simulink model "RobotX_ss_acousticsSingle_Dock_LB_ODOA_23commQualRun4pm_1025"  (R2014a)
settings: Solver=FixedStepDiscrete  StartTime=0.0  StopTime=inf  FixedStep=.25  RelTol=1e-3
undefined symbols (not defined in the file): Com1, Com2, Com3, Com4, DiscIntNeverNeededParam, standard
libraries: xpcseriallib x42, simulink x19, slrtlib x7, dspmtrx3 x2, speedgoatlib x2, speedgoatlib_IO102 x1
(part 5 of 7)

== matlab function RobotX_ss_acousticsSingle_Dock_LB_ODOA_23commQualRun4pm_1025/Main FSM/LightTower/MATLAB Function ==
  data: ltTask input; taskSelector output; pointFin input; foundInPoint input; cornerFin input; turnForSweepFin input; sweepFin input; turnForApproachFin input; approachFin input; sequenceFin input; pointEn output; cornerEn output; turnForSweepEn output; sweepEn output; turnForApproachEn output; approachEn output; sequenceEn output; reportEn output
function  [taskSelector, pointEn, cornerEn, turnForSweepEn, sweepEn, turnForApproachEn, approachEn, ...
    sequenceEn, reportEn]= ltEnabler(ltTask, pointFin, foundInPoint, ...
    cornerFin, turnForSweepFin, sweepFin, turnForApproachFin, approachFin, sequenceFin)

%%  Written by Michael Benson on October 23, 2014
%   Changes the value of ltTask and the enablers for the tasks within the
%   light tower task FSM.

%% Initialize enable signals
pointEn = 0;
cornerEn = 0;
turnForSweepEn = 0;
sweepEn = 0;
turnForApproachEn = 0;
approachEn = 0;
sequenceEn = 0;
reportEn = 0;

%% Adjust finished states based on user task selection
ltTaskStr = char(ltTask);

if ~isempty(strfind(ltTaskStr,'corner'))
    pointFin = 1;
elseif ~isempty(strfind(ltTaskStr,'sweep'))
    pointFin = 1;
    cornerFin = 1;
    turnForSweepFin = 1;
elseif ~isempty(strfind(ltTaskStr,'approach'))
    pointFin = 1;
    cornerFin = 1;
    turnForSweepFin = 1;
    sweepFin = 1;
elseif ~isempty(strfind(ltTaskStr,'sequence'))
    pointFin = 1;
    cornerFin = 1;
    turnForSweepFin = 1;
    sweepFin = 1;
    turnForApproachFin = 1;
    approachFin = 1;
elseif ~isempty(strfind(ltTaskStr,'report'))
    pointFin = 1;
    cornerFin = 1;
    turnForSweepFin = 1;
    sweepFin = 1;
    turnForApproachFin = 1;
    approachFin = 1;
    sequenceFin = 1;
end

if foundInPoint == 1
    pointFin = 1;
    cornerFin = 1;
    turnForSweepFin = 1;
    sweepFin = 1;
end
    

%% Set enable signals based on state completion
if pointFin == 0
    pointEn = 1;
    taskSelector = 1;
elseif cornerFin == 0
    cornerEn = 1;
    taskSelector = 2;
elseif turnForSweepFin == 0
    turnForSweepEn = 1;
    taskSelector = 3;
elseif sweepFin == 0
    sweepEn = 1;
    taskSelector = 4;
elseif turnForApproachFin == 0
    turnForApproachEn = 1;
    taskSelector = 5;
elseif approachFin == 0
    approachEn = 1;
    taskSelector = 6;
elseif sequenceFin == 0
    sequenceEn = 1;
    taskSelector = 7;
else
    reportEn = 1;
    taskSelector = 8;
end

== matlab function RobotX_ss_acousticsSingle_Dock_LB_ODOA_23commQualRun4pm_1025/Sensors/1025 Comms New LIDAR Mode/Message Selector/HRTLIT Message/MATLAB Function1 ==
  data: ltSeq input; LITValid output; LITSequence output
function [LITValid,LITSequence] = LITSeqParse(ltSeq)

LITValid = ltSeq(1);
LITSequence = ltSeq(2:4);

== matlab function RobotX_ss_acousticsSingle_Dock_LB_ODOA_23commQualRun4pm_1025/Sensors/1025 Comms New LIDAR Mode/Pi Nav Send/Data Update2 ==
  data: Valid input; ControlMode input; V output; C output; L output; A output; Data input; D1 output; D2 output; D3 output; D4 output; D5 output; D6 output; D7 output; D8 output; D9 output; D10 output; D11 output; D12 output; D13 output; D14 output; D15 output; D16 output; D17 output; D18 output; D19 output; D20 output; D21 output; D22 output; D23 output; D24 output; Activate input
function [V,C,L,A,D1,D2,D3,D4,D5,D6,D7,D8,D9,D10,D11,D12,D13,D14,D15,D16,D17,...
    D18,D19,D20,D21,D22,D23,D24] = dataSplit(Valid,ControlMode,Data,Activate)
%Written by Anderson Lebbad on August 10, 2014
%Last Edited by: Anderson Lebbad on September 11, 2014

%This function splits the data vector into the twelve channels it is
%composed of for communication

persistent HoldData

if isempty(HoldData)
    HoldData = zeros(26,1);
    HoldData(2) = 2;
end

if Valid == 1
    HoldData(1) = Valid;
    HoldData(2) = ControlMode;
    HoldData(3) = Data(1);
    HoldData(4) = Data(2);
    HoldData(5) = Data(3);
    HoldData(6) = Data(4);
    HoldData(7) = Data(5);
    HoldData(8) = Data(6);
    HoldData(9) = Data(7);
    HoldData(10) = Data(8);
    HoldData(11) = Data(9);
    HoldData(12) = Data(10);
    HoldData(13) = Data(11);
    HoldData(14) = Data(12);
    HoldData(15) = Data(13);
    HoldData(16) = Data(14);
    HoldData(17) = Data(15);
    HoldData(18) = Data(16);
    HoldData(19) = Data(17);
    HoldData(20) = Data(18);
    HoldData(21) = Data(19);
    HoldData(22) = Data(20);
    HoldData(23) = Data(21);
    HoldData(24) = Data(22);
    HoldData(25) = Data(23);
    HoldData(26) = Data(24);
end

V = HoldData(1);
C = HoldData(2);
L = 8;
A = Activate;
D1 = HoldData(3);
D2 = HoldData(4);
D3 = HoldData(5);
D4 = HoldData(6);
D5 = HoldData(7);
D6 = HoldData(8);
D7 = HoldData(9);
D8 = HoldData(10);
D9 = HoldData(11);
D10 = HoldData(12);
D11 = HoldData(13);
D12 = HoldData(14);
D13 = HoldData(15);
D14 = HoldData(16);
D15 = HoldData(17);
D16 = HoldData(18);
D17 = HoldData(19);
D18 = HoldData(20);
D19 = HoldData(21);
D20 = HoldData(22);
D21 = HoldData(23);
D22 = HoldData(24);
D23 = HoldData(25);
D24 = HoldData(26);

end

== matlab function RobotX_ss_acousticsSingle_Dock_LB_ODOA_23commQualRun4pm_1025/Main FSM/Docking/Docking/MATLAB Function ==
  data: QuayHeading input; TargetPoints input; Finished output; X input; Data output; Y input; Psi input; Dist input; Angles input; Prob input; Time input; dockNum input
function [Finished,Data] = Orient(QuayHeading,TargetPoints,X,Y,Psi,Dist,Angles,Prob,Time,dockNum)
%Written by Dylan DeGaetano on September 2, 2014
%Last Edited By Anderson Lebbad on September 19 2014

%This function passes the current pose data with the requrested heading
%so that the boat is facing the Quay wall.This task must be in station
%keeping mode
%
%Anderson's edit moved the orient within this function and adjusts the code
%to work better with sensing information

% 10/21 Edit: Correlates the estimated NED coord of the found symbol with
% known locations found through Ivan's map and proceeds to those locations

% Input TargetPoint is a 10x2 matrix of NED coords structured as follows
% [Observation Point; Dock1Start; Dock1Inter; Dock1Fin; Dock2Start;
% Dock2Inter; Dock2Fin; Dock3Start; Dock3Inter; Dock3Fin] where the bay
% numbers go from left to right

%work aound for communication issue
idx = Prob(4);
% Holdpose = station keeping point that we want to get to
% Pose = which waypoint to head to
% posIdx = which docking symbol position it is @
% 1 = Left, 2 = Middle, 3 = Right
% recognized = flag for if position of dock is found

persistent holdPose pos posIdx recognized

% If not to hold position
if isempty(holdPose)
    holdPose = [TargetPoints(1,:) QuayHeading]; % Initialize with Observation Points
    pos = 0;
    posIdx = 0;
    recognized = 0;
end

DistM=Dist(1)/100; % CM to M
Finished = 0; % Task not completed

%Initialize Data variable
Data = zeros(24,1); % 24x1 Array of Zeros


if idx(1) ~= 0 && recognized == 0
    %Calculate the NED coordinate of the found symbol
    TargetX = X+DistM(idx(1))*cos((Psi+Angles(idx(1)))*pi/180);
    TargetY = Y+DistM(idx(1))*sin((Psi+Angles(idx(1)))*pi/180);
    
    % Since the quay wall is very well aligned with EW directions,
    % correlate the estimated E coord of the found symbol with one of
    % the known bay positions
    bayEPos = [TargetPoints(4,2); TargetPoints(7,2); TargetPoints(10,2)];
    PosDiff = bayEPos - TargetY;
    [~,posIdx] = min(PosDiff);
    
    % Flag symbol as recognized
    recognized = 1; % Ensure that this calculation is not made again after the dock symbol pos is found/calculated
    
    % Begin proceeding to first position
    pos = 1;
end

if pos == 1
        %Set destination in front of dock to line up
        holdPose(1) = TargetPoints(pos+posIdx+2^(posIdx-1),1); % North
        holdPose(2) = TargetPoints(pos+posIdx+2^(posIdx-1),2); % East
    
    l1norm = abs(X-holdPose(1))+abs(Y-holdPose(2)); % calculate range to point we want to get to
    
    if l1norm < 2 % 2 metters
        % If within range, then flag first position complete and begin
        % proceeding to the hext position
        pos = 2;
    end
elseif pos == 2
        % Set intermediate point between start and finish
        holdPose(1) = TargetPoints(pos+posIdx+2^(posIdx-1),1); % North
        holdPose(2) = TargetPoints(pos+posIdx+2^(posIdx-1),2); % East
    
    l2norm = abs(X-holdPose(1)) + abs(Y-holdPose(2));
    
    if l2norm < 2
        % If within range, then flag second position complete and begin
        % proceeding to the hext position
        pos = 3;
    end
elseif pos == 3
        % Set final docking point
        holdPose(1) = TargetPoints(pos+posIdx+2^(posIdx-1),1); % North
        holdPose(2) = TargetPoints(pos+posIdx+2^(posIdx-1),2); % East
    
    l3norm = abs(X-holdPose(1)) + abs(Y-holdPose(2));
    
    if l3norm < 2
        holdPose = [X Y QuayHeading];
        Finished = 1;
    end
end

if Time >= 120 && recognized == 0
    % If symbol cannot be found within 60 seconds, proceed to middle bay
    posIdx = dockNum;
    recognized = 1;
end

holdPose(3) = QuayHeading;

Data(1) = holdPose(1);
Data(2) = holdPose(2);
Data(3) = holdPose(3);

== matlab function RobotX_ss_acousticsSingle_Dock_LB_ODOA_23commQualRun4pm_1025/Sensors/1020 Comms/MATLAB Function2 ==
  data: Time input; asciiLIT output; Sequence input
% This function creates the light tower message to be sent from 
% Speedgoat in ascii code
% Written by: Edward Zhu
% Date: 9/17/14

function asciiLIT = asciiLITEncoder(Time, Sequence)

% Initialize output message vector as the serial output block expects 128
% character message
asciiLIT = uint8(zeros(1,128));

% Convert static strings to ascii code
asciiMsgID = uint8('$RXLIT,');
asciiComma = uint8(',');
asciiTeamID = uint8('FAUVU,');
asciiMsgEnd = uint8('*');
asciiMsgCRLF = [13 10];

% Convert UTC Time input (hhmmss) into ascii code
asciiTime = uint8(zeros(1,7));
asciiTime(7) = asciiComma;

for timeChar = 1:6
    asciiTime(timeChar) = floor(mod(Time,10^(7-timeChar))/...
        10^(6-timeChar)) + 48;
end

% Convert the light sequece into ascii code (1 = R, 2 = B, 3 = G)
asciiSeq = uint8(zeros(1,4)+32);
asciiSeq(4) = asciiMsgEnd;

if Sequence(1) > 0 && Sequence(2) > 0 && Sequence(3) > 0
    for seqChar = 1:3
        if Sequence(seqChar) == 1
            Sequence(seqChar) = uint8('R');
        elseif Sequence(seqChar) == 2
            Sequence(seqChar) = uint8('B');
        elseif Sequence(seqChar) == 3
            Sequence(seqChar) = uint8('G');
        end
    end
    asciiSeq(1:3) = Sequence;
end

% Concat individual ascii arrays into one array
asciiPreChkSum = cat(2,asciiMsgID,asciiTime,asciiTeamID,asciiSeq);

% Calculate the checksum of the message from the '$' to the '*' and convert
% to hex
chkSum = uint8(0);

for chksumChar = 1:(length(asciiPreChkSum)-2)
    chkSum = bitxor(chkSum,asciiPreChkSum(chksumChar+1));
end

% Convert the checksum to ascii
chkSum = dec2hex(chkSum);
asciiChkSum = uint8(zeros(1,length(chkSum))+32);
for i = 1:length(chkSum)
    asciiChkSum(i) = uint8(chkSum(i));
end

% Concat the checksum and the '/r/n' to the end of the message
asciiPostChkSum = cat(2,asciiPreChkSum,asciiChkSum,asciiMsgCRLF);

% Output the final message
asciiLIT(1:length(asciiPostChkSum)) = asciiPostChkSum;

== matlab function RobotX_ss_acousticsSingle_Dock_LB_ODOA_23commQualRun4pm_1025/Main FSM/LightTower/Sweep Field/Spin, Listen, and Point/Look for Light Tower ==
  data: subsetCorners input; X input; Y input; Psi input; Distances input; Angles input; Data output; Finished output; FoundTower output; TowerLoc output; spinAmount input
function [Data, Finished, FoundTower, TowerLoc] = fcn(...
    subsetCorners, X, Y, Psi, Distances, Angles, spinAmount)

%   Written by Michael Benson on October 23, 2014
%   This function spins the WAM-V to look for the light tower.  If it
%   sees an object, and that object is within the field subset, the boat
%   will hold pose and the Lidar will continue to evaluate an object.  If
%   the object is still there within that time, it determines that that
%   object is the buoy and ends the task.  Otherwise, the task exits
%   without setting FoundTower high.

[Distances,I] = sort(Distances);
Angles = Angles(I);

persistent FoundHeading FoundCounter desiredHeading initHeading minPose maxPose minReached maxReached

offset = 5;

if isempty(FoundHeading) && isempty(FoundCounter) && isempty(desiredHeading) && isempty(initHeading) && isempty(minReached) && isempty(maxReached)
    FoundCounter = 0;
    minPose = Psi - spinAmount/2;
    maxPose = Psi + spinAmount/2;
    minReached = 0;
    maxReached = 0;
    initHeading = Psi;
    desiredHeading = Psi+offset;
    FoundHeading = 0;
end

Finished = 0;
FoundTower = 0;
Data = zeros(24,1);
TowerLoc = zeros(1,2);
LandmarkLocations = zeros(12,2);
LandmarkDistances = zeros(12,1);

ObjectInfo = [Distances,Angles];


%% Landmark Analysis
if ObjectInfo(12,1) ~= 0 && ObjectInfo(12,2) ~= 0
    %calculate location of each landmark and determine if it is in the
    %bounding box
    for i = 12-sum(Distances ~= 0)+1:12
        LandmarkX = X + cos((Psi+Angles(i))*pi/180)*Distances(i)/100;
        LandmarkY = Y + sin((Psi+Angles(i))*pi/180)*Distances(i)/100;
        LandmarkValid = inBbox(subsetCorners,[LandmarkX LandmarkY]);
        if LandmarkValid == 1
            LandmarkLocations(i,1:2) = [LandmarkX LandmarkY];
            LandmarkDistances(i) = Distances(i);
        end
    end
    
    [~,I] = sort(LandmarkDistances);
    LandmarkLocations = LandmarkLocations(I);
    
    if sum(LandmarkDistances ~= 0) >= 1
        FoundTower = 1;
        TowerLoc = LandmarkLocations(12-sum(LandmarkDistances ~= 0)+1,1:2);
        FoundCounter = FoundCounter + 1;
        if FoundCounter == 1;
            FoundHeading = Psi;
        end
        desiredHeading = FoundHeading;
    end
else
    FoundCounter = 0;
    if abs(Psi-maxPose) < 5
        maxReached = 1;
    elseif abs(Psi-minPose) < 5
        minReached = 1;
    end
    
    if maxReached == 1
        desiredHeading = Psi - offset;
    elseif maxReached == 1 && minReached == 1
        desiredHeading = initHeading;
        Finished = 1;
    end
end

Data(1:3) = [X Y desiredHeading];

end

function [ inBbox ] = inBbox( bbox, point )
%UNTITLED Summary of this function goes here
%   Detailed explanation goes here
b1 = bbox(1,:);
b2 = bbox(2,:);
b3 = bbox(3,:);
b4 = bbox(4,:);

t1 = inTriangle(point,b1,b2,b3);
t2 = inTriangle(point,b1,b2,b4);
t3 = inTriangle(point,b1,b3,b4);

if t1 && t2 && t3
    inBbox = 1;
else
    inBbox = 0;
end

end

function [ inTri ] = inTriangle(p, a, b, c)

s1 = sameSide(p,a,b,c);
s2 = sameSide(p,b,a,c);
s3 = sameSide(p,c,a,b);

if s1 || s2 || s3
    inTri = 1;
else
    inTri = 0;
end

end

function [ onSame ] = sameSide(p1,p2,a,b)

theta = atan2(b(2)-a(2),b(1)-a(1));
R = [cos(theta), sin(theta); -sin(theta), cos(theta)];
side1 = R*(p1-a)';
side2 = R*(p2-a)';
same = side1(2)/side2(2);
onSame = same >= 0;

end

== matlab function RobotX_ss_acousticsSingle_Dock_LB_ODOA_23commQualRun4pm_1025/Main FSM/LightTower/Turn For Sweep/LLA to NED ==
  data: GoalLLA input; GoalNED output; NED_origin input
function GoalNED = LLA2NEDfun(GoalLLA,NED_origin)
%Written by Anderson Lebbad on September 20, 2014
%Last edited by:
%
%This function converts a target Latitude, Longitude, Altitude (LLA) point
%into North, East, Down (NED) coordinates
GoalNED = zeros(size(GoalLLA));
for i = 1:size(GoalLLA,1)
    %First convert to earth centered, earth fixed frame
    GoalECEF = lla2ecef([GoalLLA(1)*(pi/180), GoalLLA(2)*(pi/180), 0]');
    %Then convert from ECEF to North East Down
    GoalNEDvect = ecef2ned([NED_origin(1)*(pi/180),NED_origin(2)*(pi/180)],GoalECEF);
    GoalNED(i,:) = GoalNEDvect(1:2)';
end

end

function x_ecef = lla2ecef(x_lla)
% LLE2ECEF: Converts from geodetic latitude, longitude, and altitude to earth-centered earth-fixed Cartesian coordinates
% INPUT: latitude phi (rad), longitude lambda (rad), altitude h (m)
% OUTPUT: [x, y, z]' (m) earth-centered earth-fixed Cartesian coordinates
    a = 6378137; % equatorial radius of ellipsoid (semi-major axis) (m)
    b = 6356752; % polar axis radius of ellipsoid (semi-minor axis) (m)

    phi = x_lla(1);
    lambda = x_lla(2);
    h = x_lla(3);
    
    % auxiliar quantities f, e, and N
    f = (a-b)/a;
    e = f*(2-f);
    N = a/sqrt(1-(e*sin(phi))^2);
    x_ecef = [(N+h)*cos(phi)*cos(lambda); (N+h)*cos(phi)*sin(lambda); (N*(1-e^2)+h)*sin(phi)];
end

function [x_ned] = ecef2ned(ned_lla, x_ecef)
% ECEF2NED Converts from earth-centered, earth-fixed Cartesian coordinates to tangent plane
% INPUT:
% 1) x_ecef=[x,y,z]' (m) earth-centered, earth-fixed Cartesian coordinates
% 2) ned_lla=[phi,lambda]' consiting of latitude phi (rad), longitude lambda (rad) of NED origin
% OUTPUT:
% 1) x_ned=[x,y,z]' (m) in NED coordinate system with the origin [phi,lambda]'

    phi = ned_lla(1);
    lambda = ned_lla(2);

    % transformation  matrix
    T = [-sin(phi)*cos(lambda) -sin(phi)*sin(lambda)  cos(phi)
         -sin(lambda)           cos(lambda)           0
          cos(phi)*cos(lambda)   cos(phi)*sin(lambda)  sin(phi)];

     x_ned = T*(x_ecef-lla2ecef([phi, lambda, 0]')); % convert to NED
     x_ned(3) = -x_ned(3);
end

== matlab function RobotX_ss_acousticsSingle_Dock_LB_ODOA_23commQualRun4pm_1025/Main FSM/ODOA/Entry Gate/Entry Gate Align/MATLAB Function1 ==
  data: EnterGateNED input; entryNED output; gateNumber input
function entryNED = EntryGPSSelector(EnterGateNED,gateNumber)

entryNED = EnterGateNED(gateNumber,:);

== matlab function RobotX_ss_acousticsSingle_Dock_LB_ODOA_23commQualRun4pm_1025/Main FSM/ODOA/Entry Gate/Entry Gate Enabler ==
  data: StartFin input; TaskSelector output; StartEn output; AlignFin input; AlignEn output; ThroughEn output
function [TaskSelector, StartEn,AlignEn,ThroughEn] = entryGateEnabler(StartFin, AlignFin)

StartEn = 0;
AlignEn = 0;
ThroughEn = 0;

if StartFin == 0
    StartEn = 1;
    TaskSelector = 1;
elseif AlignFin == 0
    AlignEn = 1;
    TaskSelector = 2;
else
    ThroughEn = 1;
    TaskSelector = 3;
end

== matlab function RobotX_ss_acousticsSingle_Dock_LB_ODOA_23commQualRun4pm_1025/Main FSM/ODOA/Entry Gate/Entry Gate Through/CalcTimes ==
  data: pts input; u input; Data output
function Data = calcTimes(pts, u)
%Written by Anderson Lebbad on August 9, 2014
%Last Edited: Dylan DeGaetano September 1, 2014

%Calculates times for the boat to get to points for a trajectory, and
%formats Data for communication

%Initialize
Data = zeros(24,1);
traj = zeros(8,3);
traj(:,1:2) = pts;



for k = 2:8
    %Calculate distance to travel from last point
    distTravel = sqrt(sum((pts(k-1,:)-pts(k,:)).^2));
    %Assume 1m per second speed
    traj(k,3) = traj(k-1,3) + distTravel;
    %Add time based off initial velocity to get to first point past initial
    if k == 2
        traj(k,3) = traj(k,3) + 2.5*abs(2-u);
    end
end


%Output Data
for i=1:8
    for j = 1:3
        Data(3*(i-1)+j) = traj(i,j);
    end
end

== matlab function RobotX_ss_acousticsSingle_Dock_LB_ODOA_23commQualRun4pm_1025/Main FSM/ODOA/Entry Gate/Entry Gate Through/MATLAB Function ==
  data: dist input; X input; Y input; Psi input; GoalNED output
function GoalNED = travelAlongHeading(dist, X, Y, Psi)
%Written by Michael Benson on October 23, 2014

%This function determines the target NED point for the Sweep Field subtask
%for the Light Tower task.  The target point is Distance meters from the
%current ASV position, and is towards the opposite corner of the subset
%field.

persistent lockedHeading

Psi = Psi*180/pi;

if isempty(lockedHeading)
    lockedHeading = Psi;
end

GoalNED = [X+dist*cos(lockedHeading*pi/180) Y+dist*sin(lockedHeading*pi/180)];

== matlab function RobotX_ss_acousticsSingle_Dock_LB_ODOA_23commQualRun4pm_1025/Main FSM/ODOA/Entry Gate/GPS Move/GPSMove ==
  data: GoalNED input; X input; Finished output; valid output; Y input; Psi input; pts output
function [Finished,valid,pts] = GPSmove(GoalNED,X,Y,Psi)
%Written by Dylan DeGaetano on September 1, 2014
%Last edited by: Anderson Lebbad
%
%This function will go to a given NED cooridnate, last edit changed the
%goal pt and variable names

% Input of GoalNED is a 10x2 matrix of NED coords where the first row is
% the coord of the docking observation point

persistent Sample
if isempty(Sample)
Sample = 0;
end
Finished = 0;
pts = zeros(8,2);
%$Distance to object in meters
if Sample == 100
    Sample = 0;
end

if Sample == 0
    pts(1,1) = X+5*cos(Psi*pi/180);
    pts(1,2) = Y+5*sin(Psi*pi/180);
    pts(8,1) = GoalNED(1,1);
    pts(8,2) = GoalNED(1,2);
    pts(2,:) = pts(1,:) +(1*(GoalNED(1,:)-pts(1,:))/7);
    pts(3,:) = pts(1,:) +(2*(GoalNED(1,:)-pts(1,:))/7);
    pts(4,:) = pts(1,:) +(3*(GoalNED(1,:)-pts(1,:))/7);
    pts(5,:) = pts(1,:) +(4*(GoalNED(1,:)-pts(1,:))/7);
    pts(6,:) = pts(1,:) +(5*(GoalNED(1,:)-pts(1,:))/7);
    pts(7,:) = pts(1,:) +(6*(GoalNED(1,:)-pts(1,:))/7);
    Sample = 1; 
    valid = 1;
    
else 
    range = sqrt(sum((GoalNED(1,:) - [X Y]).^2));
    if range <= 5
        Finished = 1;
    end
    valid = 0;
    Sample = Sample + 1;
end

== matlab function RobotX_ss_acousticsSingle_Dock_LB_ODOA_23commQualRun4pm_1025/Main FSM/ODOA/Exit Gate/Exit Gate Through/MATLAB Function ==
  data: dist input; X input; Y input; Psi input; GoalNED output
function GoalNED = travelAlongHeading(dist, X, Y, Psi)
%Written by Michael Benson on October 23, 2014

%This function determines the target NED point for the Sweep Field subtask
%for the Light Tower task.  The target point is Distance meters from the
%current ASV position, and is towards the opposite corner of the subset
%field.

persistent lockedHeading

Psi = Psi*180/pi;

if isempty(lockedHeading)
    lockedHeading = Psi;
end

GoalNED = [X+dist*cos(lockedHeading*pi/180) Y+dist*sin(lockedHeading*pi/180)];

== matlab function RobotX_ss_acousticsSingle_Dock_LB_ODOA_23commQualRun4pm_1025/Main FSM/ODOA/GPS Beeline/GPSMove ==
  data: dodgeStart output; GoalNED input; X input; Finished output; valid output; Y input; Psi input; pts output; Distances input
function [dodgeStart,Finished,valid,pts] = GPSmove(GoalNED,X,Y,Psi,Distances)
%Written by Dylan DeGaetano on September 1, 2014
%Last edited by: Anderson Lebbad
%
%This function will go to a given NED cooridnate, last edit changed the
%goal pt and variable names

% Input of GoalNED is a 10x2 matrix of NED coords where the first row is
% the coord of the docking observation point

DistM = Distances/100;

DistM = sort(DistM);
dodgeStart = 0;

persistent Sample
if isempty(Sample)
Sample = 0;
end
Finished = 0;
pts = zeros(8,2);
%$Distance to object in meters
if Sample == 100
    Sample = 0;
end

if Sample == 0
    pts(1,1) = X+5*cos(Psi*pi/180);
    pts(1,2) = Y+5*sin(Psi*pi/180);
    pts(8,1) = GoalNED(1,1);
    pts(8,2) = GoalNED(1,2);
    pts(2,:) = pts(1,:) +(1*(GoalNED(1,:)-pts(1,:))/7);
    pts(3,:) = pts(1,:) +(2*(GoalNED(1,:)-pts(1,:))/7);
    pts(4,:) = pts(1,:) +(3*(GoalNED(1,:)-pts(1,:))/7);
    pts(5,:) = pts(1,:) +(4*(GoalNED(1,:)-pts(1,:))/7);
    pts(6,:) = pts(1,:) +(5*(GoalNED(1,:)-pts(1,:))/7);
    pts(7,:) = pts(1,:) +(6*(GoalNED(1,:)-pts(1,:))/7);
    Sample = 1; 
    valid = 1;
    
else 
    range = sqrt(sum((GoalNED(1,:) - [X Y]).^2));
    if range <= 5
        Finished = 1;
    end
    valid = 0;
    Sample = Sample + 1;
end

if sum(DistM ~= 0) > 0
    closestRange = DistM(12-sum(DistM ~= 0)+1);
    if closestRange < 10
        dodgeStart = 1;
    end
end

== matlab function RobotX_ss_acousticsSingle_Dock_LB_ODOA_23commQualRun4pm_1025/Main FSM/Start//Speedgate/GPS Move/CalcTimes ==
  data: pts input; u input; Data output
function Data = calcTimes(pts, u)
%Written by Anderson Lebbad on August 9, 2014
%Last Edited: Dylan DeGaetano September 1, 2014

%Calculates times for the boat to get to points for a trajectory, and
%formats Data for communication

%Initialize
Data = zeros(24,1);
traj = zeros(8,3);
traj(:,1:2) = pts;



for k = 2:8
    %Calculate distance to travel from last point
    distTravel = sqrt(sum((pts(k-1,:)-pts(k,:)).^2));
    %Assume 1m per second speed
    traj(k,3) = traj(k-1,3) + distTravel;
    %Add time based off initial velocity to get to first point past initial
    if k == 2
        traj(k,3) = traj(k,3) + 2.5*abs(2-u);
    end
end


%Output Data
for i=1:8
    for j = 1:3
        Data(3*(i-1)+j) = traj(i,j);
    end
end

== matlab function RobotX_ss_acousticsSingle_Dock_LB_ODOA_23commQualRun4pm_1025/Main FSM/Start//Speedgate/Main Enabler ==
  data: taskSelector output; GpsEn output; entEn output; exitEn output; ssgateTask input; GpsFin input; entFin input
function [taskSelector,GpsEn,entEn,exitEn]=Startgate_Enabler(ssgateTask,...
    GpsFin,entFin)
%Written by Anderson Lebbad on July 19, 2013
%Last Edited: Dylan DeGaetano on September ,4 2014
%   Substring search for task was written in
%   Case switches were redundant, combined with first set of if statements

%Changes the value of MainMode and the enablers for the tasks within the
%Main FSM.

% Initialize enable signals
GpsEn = 0;
entEn =0;
exitEn = 0;

% Convert main task indicator to a string
ssgateTaskStr = char(ssgateTask);

% Adjust finished states based on user task selection (never skips
% initialization)
if ~isempty(strfind(ssgateTaskStr,'Aim'))
    GpsFin = 1;
elseif ~isempty(strfind(ssgateTaskStr,'Start'))
    GpsFin = 1;
    entFin = 1;
elseif ~isempty(strfind(ssgateTaskStr,'Speed'))
    GpsFin = 1;
    entFin = 1;
end

% Set enable signals based on state completion
if GpsFin == 0
    GpsEn = 1;
    taskSelector = 1;
elseif entFin == 0
    entEn = 1;
    taskSelector = 2;
else
    exitEn = 1;
    taskSelector = 3;
end

== system RobotX_ss_acousticsSingle_Dock_LB_ODOA_23commQualRun4pm_1025/Main FSM/ODOA/Entry Gate/Entry Gate Align ==
  Sensors : Inport
  Enable : EnablePort  ShowOutputPort=on
  Bus Selector : BusSelector  OutputSignals=Navigation Message.Pose.X,Navigation Message.Pose.Y,Navigation Message.Pose.Psi,Lidar Data Input.Landmarks.Distances,Lidar Data Input.Landmarks.Angles
  Compare To Constant : simulink/Logic and Bit Operations/Compare To Constant  relop=>=  const=120  OutDataTypeStr=boolean
  Data Store Read : DataStoreRead  DataStoreName=EnterGateNED
  Data Store Read1 : DataStoreRead  DataStoreName=ODOAentry
  Data Store Read2 : DataStoreRead  DataStoreName=QuayHeading
  Data Store Read3 : DataStoreRead  DataStoreName=ODOAstartNED
  Data Type Conversion : DataTypeConversion  OutDataTypeStr=double
  Discrete-Time Integrator : DiscreteIntegrator  SampleTime=-1  ICPrevOutput=DiscIntNeverNeededParam  ICPrevScaledInput=DiscIntNeverNeededParam
  Logical Operator : Logic  Operator=OR  AllPortsSameDT=off  OutDataTypeStr=boolean
  MATLAB Function : MATLAB Function  TreatAsAtomicUnit=on
  MATLAB Function1 : MATLAB Function  TreatAsAtomicUnit=on
  Output Heirarchy : Subsystem
  Outputs : Outport
  Finished : Outport  Port=2
  wires:
  Output Heirarchy/1(Outputs) -> Outputs/1
  Sensors/1 -> Output Heirarchy/2(Sensors), Bus Selector/1
  Data Store Read1/1 -> MATLAB Function1/2(gateNumber)
  Data Store Read/1 -> MATLAB Function1/1(EnterGateNED)
  MATLAB Function1/1(entryNED) -> MATLAB Function/1(entryNED)
  Bus Selector/1 -> MATLAB Function/5(X)  "<X>"
  Bus Selector/5 -> MATLAB Function/9(Angles)  "<Angles>"
  Bus Selector/2 -> MATLAB Function/6(Y)  "<Y>"
  Bus Selector/4 -> MATLAB Function/8(Distances)  "<Distances>"
  Bus Selector/3 -> MATLAB Function/7(Psi)  "<Psi>"
  MATLAB Function/2(Finished) -> Logical Operator/1
  MATLAB Function/1(Data) -> Output Heirarchy/1(Data)
  Discrete-Time Integrator/1 -> Compare To Constant/1, MATLAB Function/4(Time)
  Enable/1 -> Discrete-Time Integrator/1
  Data Store Read2/1 -> MATLAB Function/3(QuayHeading)
  Data Store Read3/1 -> MATLAB Function/2(startNED)
  Compare To Constant/1 -> Logical Operator/2
  Logical Operator/1 -> Data Type Conversion/1
  Data Type Conversion/1 -> Finished/1

== system RobotX_ss_acousticsSingle_Dock_LB_ODOA_23commQualRun4pm_1025/Main FSM/ODOA/Entry Gate/Entry Gate Through ==
  Sensors : Inport
  Enable : EnablePort
  Bus Selector : BusSelector  OutputSignals=Navigation Message.Pose.X,Navigation Message.Pose.Y,Navigation Message.Pose.Psi,Navigation Message.Velocity.u
  CalcTimes : MATLAB Function  TreatAsAtomicUnit=on
  Distance to Travel : Constant  Value=15
  GPSMove : MATLAB Function  TreatAsAtomicUnit=on
  MATLAB Function : MATLAB Function  TreatAsAtomicUnit=on
  Output Reassign : Subsystem
  Outputs : Outport
  Finished : Outport  Port=2
  wires:
  GPSMove/3(pts) -> CalcTimes/1(pts)
  Sensors/1 -> Output Reassign/3(Sensors), Bus Selector/1
  Bus Selector/1 -> MATLAB Function/2(X), GPSMove/2(X)  "<X>"
  Bus Selector/2 -> MATLAB Function/3(Y), GPSMove/3(Y)  "<Y>"
  Bus Selector/3 -> MATLAB Function/4(Psi), GPSMove/4(Psi)  "<Psi>"
  Bus Selector/4 -> CalcTimes/2(u)  "<u>"
  GPSMove/1(Finished) -> Finished/1
  Output Reassign/1(Outputs) -> Outputs/1
  CalcTimes/1(Data) -> Output Reassign/2(Data)
  GPSMove/2(valid) -> Output Reassign/1(Vaild)
  MATLAB Function/1(GoalNED) -> GPSMove/1(GoalNED)
  Distance to Travel/1 -> MATLAB Function/1(dist)

== system RobotX_ss_acousticsSingle_Dock_LB_ODOA_23commQualRun4pm_1025/Main FSM/ODOA/Entry Gate/GPS Move ==
  Sensors : Inport
  Enable : EnablePort
  Bus Selector : BusSelector  OutputSignals=Navigation Message.Pose.X,Navigation Message.Pose.Y,Navigation Message.Pose.Psi,Navigation Message.Velocity.u
  CalcTimes : MATLAB Function  TreatAsAtomicUnit=on
  Data Store Read : DataStoreRead  DataStoreName=EnterGateNED
  Data Store Read1 : DataStoreRead  DataStoreName=ODOAentry
  GPSMove : MATLAB Function  TreatAsAtomicUnit=on
  MATLAB Function1 : MATLAB Function  TreatAsAtomicUnit=on
  Output Reassign : Subsystem
  Outputs : Outport
  Finished : Outport  Port=2
  wires:
  GPSMove/3(pts) -> CalcTimes/1(pts)
  Sensors/1 -> Output Reassign/3(Sensors), Bus Selector/1
  Bus Selector/1 -> GPSMove/2(X)  "<X>"
  Bus Selector/2 -> GPSMove/3(Y)  "<Y>"
  Bus Selector/3 -> GPSMove/4(Psi)  "<Psi>"
  Bus Selector/4 -> CalcTimes/2(u)  "<u>"
  GPSMove/1(Finished) -> Finished/1
  Output Reassign/1(Outputs) -> Outputs/1
  CalcTimes/1(Data) -> Output Reassign/2(Data)
  GPSMove/2(valid) -> Output Reassign/1(Vaild)
  MATLAB Function1/1(entryGPS) -> GPSMove/1(GoalNED)
  Data Store Read1/1 -> MATLAB Function1/2(gateNumber)
  Data Store Read/1 -> MATLAB Function1/1(EnterGateGPS)

== system RobotX_ss_acousticsSingle_Dock_LB_ODOA_23commQualRun4pm_1025/Main FSM/ODOA/Exit Gate/Exit Gate Align ==
  Sensors : Inport
  Enable : EnablePort  ShowOutputPort=on
  Bus Selector : BusSelector  OutputSignals=Navigation Message.Pose.X,Navigation Message.Pose.Y,Navigation Message.Pose.Psi,Lidar Data Input.Landmarks.Distances,Lidar Data Input.Landmarks.Angles
  Compare To Constant : simulink/Logic and Bit Operations/Compare To Constant  relop=>=  const=120  OutDataTypeStr=boolean
  Data Store Read2 : DataStoreRead  DataStoreName=QuayHeading
  Data Type Conversion : DataTypeConversion  OutDataTypeStr=double
  Discrete-Time Integrator : DiscreteIntegrator  SampleTime=-1  ICPrevOutput=DiscIntNeverNeededParam  ICPrevScaledInput=DiscIntNeverNeededParam
  Logical Operator : Logic  Operator=OR  AllPortsSameDT=off  OutDataTypeStr=boolean
  MATLAB Function : MATLAB Function  TreatAsAtomicUnit=on
  Output Heirarchy : Subsystem
  Outputs : Outport
  Finished : Outport  Port=2
  wires:
  Output Heirarchy/1(Outputs) -> Outputs/1
  Sensors/1 -> Output Heirarchy/2(Sensors), Bus Selector/1
  Bus Selector/1 -> MATLAB Function/3(X)  "<X>"
  Bus Selector/5 -> MATLAB Function/7(Angles)  "<Angles>"
  Bus Selector/2 -> MATLAB Function/4(Y)  "<Y>"
  Bus Selector/4 -> MATLAB Function/6(Distances)  "<Distances>"
  Bus Selector/3 -> MATLAB Function/5(Psi)  "<Psi>"
  MATLAB Function/2(Finished) -> Logical Operator/1
  MATLAB Function/1(Data) -> Output Heirarchy/1(Data)
  Discrete-Time Integrator/1 -> Compare To Constant/1, MATLAB Function/2(Time)
  Enable/1 -> Discrete-Time Integrator/1
  Data Store Read2/1 -> MATLAB Function/1(QuayHeading)
  Compare To Constant/1 -> Logical Operator/2
  Logical Operator/1 -> Data Type Conversion/1
  Data Type Conversion/1 -> Finished/1

== system RobotX_ss_acousticsSingle_Dock_LB_ODOA_23commQualRun4pm_1025/Main FSM/ODOA/Exit Gate/Exit Gate Through ==
  Sensors : Inport
  Enable : EnablePort
  Bus Selector : BusSelector  OutputSignals=Navigation Message.Pose.X,Navigation Message.Pose.Y,Navigation Message.Pose.Psi,Navigation Message.Velocity.u
  CalcTimes : MATLAB Function  TreatAsAtomicUnit=on
  Distance to Travel : Constant  Value=15
  GPSMove : MATLAB Function  TreatAsAtomicUnit=on
  MATLAB Function : MATLAB Function  TreatAsAtomicUnit=on
  Output Reassign : Subsystem
  Outputs : Outport
  Finished : Outport  Port=2
  wires:
  GPSMove/3(pts) -> CalcTimes/1(pts)
  Sensors/1 -> Output Reassign/3(Sensors), Bus Selector/1
  Bus Selector/1 -> MATLAB Function/2(X), GPSMove/2(X)  "<X>"
  Bus Selector/2 -> MATLAB Function/3(Y), GPSMove/3(Y)  "<Y>"
  Bus Selector/3 -> MATLAB Function/4(Psi), GPSMove/4(Psi)  "<Psi>"
  Bus Selector/4 -> CalcTimes/2(u)  "<u>"
  GPSMove/1(Finished) -> Finished/1
  Output Reassign/1(Outputs) -> Outputs/1
  CalcTimes/1(Data) -> Output Reassign/2(Data)
  GPSMove/2(valid) -> Output Reassign/1(Vaild)
  MATLAB Function/1(GoalNED) -> GPSMove/1(GoalNED)
  Distance to Travel/1 -> MATLAB Function/1(dist)

== system RobotX_ss_acousticsSingle_Dock_LB_ODOA_23commQualRun4pm_1025/Main FSM/ODOA/GPS Beeline/Output Reassign ==
  Vaild : Inport
  Data : Inport  Port=2
  Sensors : Inport  Port=3
  Acoustic Active : Constant  Value=0
  Bus Creator2 : BusCreator  Inputs=3
  Bus Creator3 : BusCreator  Inputs=3
  Bus Creator5 : BusCreator  Inputs=2
  Constant3 : Constant  Value=0
  Lidar Mode : Constant  Value=7
  Outputs : Outport
  wires:
  Sensors/1 -> Bus Creator5/2  "Sensors"
  Bus Creator5/1 -> Outputs/1  "Output Signals"
  Vaild/1 -> Bus Creator2/1  "Valid"
  Constant3/1 -> Bus Creator2/2  "Control Mode"
  Data/1 -> Bus Creator2/3  "Data"
  Bus Creator2/1 -> Bus Creator3/1  "Navigation Outputs"
  Acoustic Active/1 -> Bus Creator3/2  "Acoustic Active"
  Lidar Mode/1 -> Bus Creator3/3  "Lidar Mode"
  Bus Creator3/1 -> Bus Creator5/1  "Outputs"

== system RobotX_ss_acousticsSingle_Dock_LB_ODOA_23commQualRun4pm_1025/Main FSM/Start//Speedgate/Aim/Output Heirarchy ==
  Data : Inport
  Sensors : Inport  Port=2
  Acoustic Active : Constant  Value=0
  Bus Creator2 : BusCreator  Inputs=3
  Bus Creator3 : BusCreator  Inputs=3
  Bus Creator5 : BusCreator  Inputs=2
  Constant : Constant
  Constant3 : Constant
  Lidar Mode : Constant
  Outputs : Outport
  wires:
  Sensors/1 -> Bus Creator5/2  "Sensors"
  Bus Creator5/1 -> Outputs/1  "Output Signals"
  Constant/1 -> Bus Creator2/1  "Valid"
  Constant3/1 -> Bus Creator2/2  "Control Mode"
  Data/1 -> Bus Creator2/3  "Data"
  Bus Creator2/1 -> Bus Creator3/1  "Navigation Outputs"
  Acoustic Active/1 -> Bus Creator3/2  "Acoustic Active"
  Lidar Mode/1 -> Bus Creator3/3  "Lidar Mode"
  Bus Creator3/1 -> Bus Creator5/1  "Outputs"

== system RobotX_ss_acousticsSingle_Dock_LB_ODOA_23commQualRun4pm_1025/Main FSM/Start//Speedgate/Dead Reckon/Output Reassign ==
  Vaild : Inport
  Data : Inport  Port=2
  Sensors : Inport  Port=3
  Acoustic Active : Constant  Value=0
  Bus Creator2 : BusCreator  Inputs=3
  Bus Creator3 : BusCreator  Inputs=3
  Bus Creator5 : BusCreator  Inputs=2
  Constant3 : Constant  Value=0
  Lidar Mode : Constant  Value=3
  Outputs : Outport
  wires:
  Sensors/1 -> Bus Creator5/2  "Sensors"
  Bus Creator5/1 -> Outputs/1  "Output Signals"
  Vaild/1 -> Bus Creator2/1  "Valid"
  Constant3/1 -> Bus Creator2/2  "Control Mode"
  Data/1 -> Bus Creator2/3  "Data"
  Bus Creator2/1 -> Bus Creator3/1  "Navigation Outputs"
  Acoustic Active/1 -> Bus Creator3/2  "Acoustic Active"
  Lidar Mode/1 -> Bus Creator3/3  "Lidar Mode"
  Bus Creator3/1 -> Bus Creator5/1  "Outputs"

== system RobotX_ss_acousticsSingle_Dock_LB_ODOA_23commQualRun4pm_1025/Main FSM/Start//Speedgate/GPS Move/Output Reassign ==
  Vaild : Inport
  Data : Inport  Port=2
  Sensors : Inport  Port=3
  Acoustic Active : Constant  Value=0
  Bus Creator2 : BusCreator  Inputs=3
  Bus Creator3 : BusCreator  Inputs=3
  Bus Creator5 : BusCreator  Inputs=2
  Constant3 : Constant  Value=0
  Lidar Mode : Constant  Value=0
  Outputs : Outport
  wires:
  Sensors/1 -> Bus Creator5/2  "Sensors"
  Bus Creator5/1 -> Outputs/1  "Output Signals"
  Vaild/1 -> Bus Creator2/1  "Valid"
  Constant3/1 -> Bus Creator2/2  "Control Mode"
  Data/1 -> Bus Creator2/3  "Data"
  Bus Creator2/1 -> Bus Creator3/1  "Navigation Outputs"
  Acoustic Active/1 -> Bus Creator3/2  "Acoustic Active"
  Lidar Mode/1 -> Bus Creator3/3  "Lidar Mode"
  Bus Creator3/1 -> Bus Creator5/1  "Outputs"

== system RobotX_ss_acousticsSingle_Dock_LB_ODOA_23commQualRun4pm_1025/Sensors/1025 Comms New LIDAR Mode/Message Selector/HRT Message ==
  Parameters : Inport
  Time : Inport  Port=2
  Bus Selector : BusSelector  OutputSignals=Sensors.Navigation Message.GPS (LLA).Lat,Sensors.Navigation Message.GPS (LLA).Long,Sensors.Navigation Message.On/Off/RC/Auto,Main Task
  MATLAB Function : MATLAB Function  TreatAsAtomicUnit=on
  HRT Message : Outport
  wires:
  MATLAB Function/1(asciiHRT) -> HRT Message/1
  Parameters/1 -> Bus Selector/1
  Time/1 -> MATLAB Function/1(Time)
  Bus Selector/1 -> MATLAB Function/2(HRTLat)  "<Lat>"
  Bus Selector/2 -> MATLAB Function/3(HRTLong)  "<Long>"
  Bus Selector/3 -> MATLAB Function/4(HRTMode)  "<On/Off/RC/Auto>"
  Bus Selector/4 -> MATLAB Function/5(HRTTask)  "<Main Task>"

== system RobotX_ss_acousticsSingle_Dock_LB_ODOA_23commQualRun4pm_1025/Sensors/1025 Comms New LIDAR Mode/Message Selector/HRTLIT Message ==
  Parameters : Inport
  Time : Inport  Port=2
  Bus Selector : BusSelector  OutputSignals=Sensors.Navigation Message.GPS (LLA).Lat,Sensors.Navigation Message.GPS (LLA).Long,Main Task,Sensors.Navigation Message.On/Off/RC/Auto
  Data Store Read1 : DataStoreRead  DataStoreName=ltSeq
  MATLAB Function : MATLAB Function  TreatAsAtomicUnit=on
  MATLAB Function1 : MATLAB Function  TreatAsAtomicUnit=on
  HRTLIT Message : Outport
  wires:
  MATLAB Function/1(asciiHRTLIT) -> HRTLIT Message/1
  Time/1 -> MATLAB Function/1(Time)
  Parameters/1 -> Bus Selector/1
  Bus Selector/3 -> MATLAB Function/4(HRTTask)  "<Main Task>"
  Bus Selector/2 -> MATLAB Function/3(HRTLong)  "<Long>"
  Bus Selector/1 -> MATLAB Function/2(HRTLat)  "<Lat>"
  Bus Selector/4 -> MATLAB Function/5(HRTMode)  "<On/Off/RC/Auto>"
  Data Store Read1/1 -> MATLAB Function1/1(ltSeq)
  MATLAB Function1/2(LITSequence) -> MATLAB Function/7(LITSequence)
  MATLAB Function1/1(LITValid) -> MATLAB Function/6(LITValid)

== system RobotX_ss_acousticsSingle_Dock_LB_ODOA_23commQualRun4pm_1025/Sensors/1025 Comms New LIDAR Mode/Message Selector/HRTSEA Message ==
  Parameters : Inport
  Time : Inport  Port=2
  Bus Selector : BusSelector  OutputSignals=Sensors.Navigation Message.GPS (LLA).Lat,Sensors.Navigation Message.GPS (LLA).Long,Main Task,Sensors.Navigation Message.On/Off/RC/Auto
  Data Store Read3 : DataStoreRead  DataStoreName=pingerInfo
  MATLAB Function : MATLAB Function  TreatAsAtomicUnit=on
  MATLAB Function1 : MATLAB Function  TreatAsAtomicUnit=on
  HRTSEA Message : Outport
  wires:
  MATLAB Function/1(asciiHRTSEA) -> HRTSEA Message/1
  Parameters/1 -> Bus Selector/1
  Time/1 -> MATLAB Function/1(Time)
  Data Store Read3/1 -> MATLAB Function1/1(pingerInfo)
  Bus Selector/3 -> MATLAB Function/4(HRTTask)  "<Main Task>"
  Bus Selector/1 -> MATLAB Function/2(HRTLat)  "<Lat>"
  Bus Selector/2 -> MATLAB Function/3(HRTLong)  "<Long>"
  Bus Selector/4 -> MATLAB Function/5(HRTMode)  "<On/Off/RC/Auto>"
  MATLAB Function1/3(SEALong) -> MATLAB Function/8(SEALong)
  MATLAB Function1/2(SEALat) -> MATLAB Function/7(SEALat)
  MATLAB Function1/5(SEADepth) -> MATLAB Function/10(SEADepth)
  MATLAB Function1/4(SEAColor) -> MATLAB Function/9(SEAColor)
  MATLAB Function1/1(SEAValid) -> MATLAB Function/6(SEAValid)

== system RobotX_ss_acousticsSingle_Dock_LB_ODOA_23commQualRun4pm_1025/Main FSM/LightTower/Sweep Field/Drive to Point/Output Reassign ==
  Vaild : Inport
  Data : Inport  Port=2
  Sensors : Inport  Port=3
  Acoustic Active : Constant  Value=0
  Bus Creator2 : BusCreator  Inputs=3
  Bus Creator3 : BusCreator  Inputs=3
  Bus Creator5 : BusCreator  Inputs=2
  Constant3 : Constant  Value=0
  Lidar Mode : Constant  Value=7
  Outputs : Outport
  wires:
  Sensors/1 -> Bus Creator5/2  "Sensors"
  Bus Creator5/1 -> Outputs/1  "Output Signals"
  Vaild/1 -> Bus Creator2/1  "Valid"
  Constant3/1 -> Bus Creator2/2  "Control Mode"
  Data/1 -> Bus Creator2/3  "Data"
  Bus Creator2/1 -> Bus Creator3/1  "Navigation Outputs"
  Acoustic Active/1 -> Bus Creator3/2  "Acoustic Active"
  Lidar Mode/1 -> Bus Creator3/3  "Lidar Mode"
  Bus Creator3/1 -> Bus Creator5/1  "Outputs"

== system RobotX_ss_acousticsSingle_Dock_LB_ODOA_23commQualRun4pm_1025/Main FSM/LightTower/Sweep Field/Spin, Listen, and Point/Output Reassign1 ==
  Data : Inport
  Sensors : Inport  Port=2
  Acoustic Active : Constant  Value=0
  Bus Creator2 : BusCreator  Inputs=3
  Bus Creator3 : BusCreator  Inputs=3
  Bus Creator5 : BusCreator  Inputs=2
  Constant1 : Constant
  Constant3 : Constant
  Lidar Mode : Constant  Value=7
  Outputs : Outport
  wires:
  Sensors/1 -> Bus Creator5/2  "Sensors"
  Bus Creator5/1 -> Outputs/1  "Output Signals"
  Constant1/1 -> Bus Creator2/1  "Valid"
  Constant3/1 -> Bus Creator2/2  "Control Mode"
  Data/1 -> Bus Creator2/3  "Data"
  Bus Creator2/1 -> Bus Creator3/1  "Navigation Outputs"
  Acoustic Active/1 -> Bus Creator3/2  "Acoustic Active"
  Lidar Mode/1 -> Bus Creator3/3  "Lidar Mode"
  Bus Creator3/1 -> Bus Creator5/1  "Outputs"

== system RobotX_ss_acousticsSingle_Dock_LB_ODOA_23commQualRun4pm_1025/Main FSM/ODOA/Entry Gate/Entry Gate Align/Output Heirarchy ==
  Data : Inport
  Sensors : Inport  Port=2
  Acoustic Active : Constant  Value=0
  Bus Creator2 : BusCreator  Inputs=3
  Bus Creator3 : BusCreator  Inputs=3
  Bus Creator5 : BusCreator  Inputs=2
  Constant : Constant
  Constant1 : Constant
  Lidar Mode : Constant  Value=7
  Outputs : Outport
  wires:
  Sensors/1 -> Bus Creator5/2  "Sensors"
  Bus Creator5/1 -> Outputs/1  "Output Signals"
  Constant/1 -> Bus Creator2/1  "Valid"
  Constant1/1 -> Bus Creator2/2  "Control Mode"
  Data/1 -> Bus Creator2/3  "Data"
  Bus Creator2/1 -> Bus Creator3/1  "Navigation Outputs"
  Acoustic Active/1 -> Bus Creator3/2  "Acoustic Active"
  Lidar Mode/1 -> Bus Creator3/3  "Lidar Mode"
  Bus Creator3/1 -> Bus Creator5/1  "Outputs"

== system RobotX_ss_acousticsSingle_Dock_LB_ODOA_23commQualRun4pm_1025/Main FSM/ODOA/Entry Gate/Entry Gate Through/Output Reassign ==
  Vaild : Inport
  Data : Inport  Port=2
  Sensors : Inport  Port=3
  Acoustic Active : Constant  Value=0
  Bus Creator2 : BusCreator  Inputs=3
  Bus Creator3 : BusCreator  Inputs=3
  Bus Creator5 : BusCreator  Inputs=2
  Constant3 : Constant  Value=0
  Lidar Mode : Constant  Value=7
  Outputs : Outport
  wires:
  Sensors/1 -> Bus Creator5/2  "Sensors"
  Bus Creator5/1 -> Outputs/1  "Output Signals"
  Vaild/1 -> Bus Creator2/1  "Valid"
  Constant3/1 -> Bus Creator2/2  "Control Mode"
  Data/1 -> Bus Creator2/3  "Data"
  Bus Creator2/1 -> Bus Creator3/1  "Navigation Outputs"
  Acoustic Active/1 -> Bus Creator3/2  "Acoustic Active"
  Lidar Mode/1 -> Bus Creator3/3  "Lidar Mode"
  Bus Creator3/1 -> Bus Creator5/1  "Outputs"

== system RobotX_ss_acousticsSingle_Dock_LB_ODOA_23commQualRun4pm_1025/Main FSM/ODOA/Entry Gate/GPS Move/Output Reassign ==
  Vaild : Inport
  Data : Inport  Port=2
  Sensors : Inport  Port=3
  Acoustic Active : Constant  Value=0
  Bus Creator2 : BusCreator  Inputs=3
  Bus Creator3 : BusCreator  Inputs=3
  Bus Creator5 : BusCreator  Inputs=2
  Constant3 : Constant  Value=0
  Lidar Mode : Constant  Value=7
  Outputs : Outport
  wires:
  Sensors/1 -> Bus Creator5/2  "Sensors"
  Bus Creator5/1 -> Outputs/1  "Output Signals"
  Vaild/1 -> Bus Creator2/1  "Valid"
  Constant3/1 -> Bus Creator2/2  "Control Mode"
  Data/1 -> Bus Creator2/3  "Data"
  Bus Creator2/1 -> Bus Creator3/1  "Navigation Outputs"
  Acoustic Active/1 -> Bus Creator3/2  "Acoustic Active"
  Lidar Mode/1 -> Bus Creator3/3  "Lidar Mode"
  Bus Creator3/1 -> Bus Creator5/1  "Outputs"

== system RobotX_ss_acousticsSingle_Dock_LB_ODOA_23commQualRun4pm_1025/Main FSM/ODOA/Exit Gate/Exit Gate Align/Output Heirarchy ==
  Data : Inport
  Sensors : Inport  Port=2
  Acoustic Active : Constant  Value=0
  Bus Creator2 : BusCreator  Inputs=3
  Bus Creator3 : BusCreator  Inputs=3
  Bus Creator5 : BusCreator  Inputs=2
  Constant : Constant
  Constant1 : Constant
  Lidar Mode : Constant  Value=7
  Outputs : Outport
  wires:
  Sensors/1 -> Bus Creator5/2  "Sensors"
  Bus Creator5/1 -> Outputs/1  "Output Signals"
  Constant/1 -> Bus Creator2/1  "Valid"
  Constant1/1 -> Bus Creator2/2  "Control Mode"
  Data/1 -> Bus Creator2/3  "Data"
  Bus Creator2/1 -> Bus Creator3/1  "Navigation Outputs"
  Acoustic Active/1 -> Bus Creator3/2  "Acoustic Active"
  Lidar Mode/1 -> Bus Creator3/3  "Lidar Mode"
  Bus Creator3/1 -> Bus Creator5/1  "Outputs"

== system RobotX_ss_acousticsSingle_Dock_LB_ODOA_23commQualRun4pm_1025/Main FSM/ODOA/Exit Gate/Exit Gate Through/Output Reassign ==
  Vaild : Inport
  Data : Inport  Port=2
  Sensors : Inport  Port=3
  Acoustic Active : Constant  Value=0
  Bus Creator2 : BusCreator  Inputs=3
  Bus Creator3 : BusCreator  Inputs=3
  Bus Creator5 : BusCreator  Inputs=2
  Constant3 : Constant  Value=0
  Lidar Mode : Constant  Value=7
  Outputs : Outport
  wires:
  Sensors/1 -> Bus Creator5/2  "Sensors"
  Bus Creator5/1 -> Outputs/1  "Output Signals"
  Vaild/1 -> Bus Creator2/1  "Valid"
  Constant3/1 -> Bus Creator2/2  "Control Mode"
  Data/1 -> Bus Creator2/3  "Data"
  Bus Creator2/1 -> Bus Creator3/1  "Navigation Outputs"
  Acoustic Active/1 -> Bus Creator3/2  "Acoustic Active"
  Lidar Mode/1 -> Bus Creator3/3  "Lidar Mode"
  Bus Creator3/1 -> Bus Creator5/1  "Outputs"

== matlab function RobotX_ss_acousticsSingle_Dock_LB_ODOA_23commQualRun4pm_1025/Main FSM/Acoustic Single Point FSM/Report/writePingInfo ==
  data: acouX input; acouY input; Depth input; NED_Origin input; pingerInfo output; AcousticPose1 input; colorQuad input
function pingerInfo = writePingInfo(acouX,acouY,Depth,NED_Origin,AcousticPose1,colorQuad)
%Written By Anderson Lebbad on October 22, 2014
%Last Edited By:
%
%This function takes the info from the acoustic pose to create an estimate
%of pinger position in North East Down coordinates, then converts that to
%LLA. From here, a buoy color is chosen based off the quadrant, and the
%info is formatted for the message writing block - including the valid bit.

Psi = AcousticPose1(3);

%Quadrants -
%NE : 1
%SE : 2
%SW : 3
%NW : 4
Quad = round((mod(Psi,360)+45)/90);



%Color code-
%R : 1
%G : 2
%B : 3
%W : 4
%K : 5

switch Quad
    case 1
        color = colorQuad(1);
    case 2
        color = colorQuad(2);
    case 3
        color = colorQuad(3);
    otherwise
        color = colorQuad(4);
end

%Convert to LLA
LLA = ecef2lla(ned2ecef(NED_Origin'*pi/180,[acouX; acouY; 0]))*180/pi;

%Output
pingerInfo = [1, LLA(1), LLA(2), Depth, color];

end

function x_ecef = ned2ecef(ned_lla, x_ned)
% NED2ECEF 
% INPUT:
% 1) x_ned=[x,y,z]' (m) NED coordinates
% 2) ned_lla=[phi,lambda]' consiting of latitude phi (rad) and longitude lambda (rad) of NED origin
% OUTPUT:
% 1) x_ecef=[x,y,z]' (m) in earth-centered, earth-fixed coordinate system with the origin [phi,lambda]'

    phi = ned_lla(1);
    lambda = ned_lla(2);

    % transformation  matrix
    T = [-sin(phi)*cos(lambda) -sin(phi)*sin(lambda)  cos(phi)
         -sin(lambda)           cos(lambda)           0
          cos(phi)*cos(lambda)   cos(phi)*sin(lambda)  sin(phi)];
    
    x_ecef = T'*x_ned + lla2ecef([phi, lambda, 0]');
end

function [x_lla] = ecef2lla(x_ecef)
% ECEF2LLH Converts from earth-centered, earth-fixed Cartesian coordinates to latitude, longitude, and altitude
% INPUT: x_ecef=[x,y,z]' (m) earth-centered, earth-fixed Cartesian coordinates
% OUTPUT: x_lla=[phi, lambda, h]' (rad, rad, m) GPS coordinates
    a = 6378137; % equatorial radius of ellipsoid (semi-major axis) (m)
    b = 6356752; % polar axis radius of ellipsoid (semi-minor axis) (m)

    x = x_ecef(1);
    y = x_ecef(2);
    z = x_ecef(3);
    
    % define auxiliary parameters e and f
    f = (a-b)/a;
    e = f*(2-f);
    
    lambda = atan2(y,x);
    phi = atan2(inv(1-e^2)*z,sqrt(x^2+y^2));
    N = a/sqrt(1-(e*sin(phi))^2);
    h = sqrt(x^2+y^2)/cos(phi)-N;
    
    x_lla = [phi; lambda; h];
end
